simulink model "Sim_exercise2"  (R2016a)
settings: Solver=ode45  SolverMode=SingleTasking  StartTime=0.0  StopTime=10.0  RelTol=1e-3
values from neighbouring files (symbols this model uses):
  A = [-R/L 0 -Kemf/L; 0 0 1; Km/Jeq 0 -dm/Jeq]    [Exercise_1.m]    (also in Exercise_3.m = [0 1; 0 -(dm/Jeq + Km*Kemf/(R*Jeq))])
  B = [1/L; 0; 0]    [Exercise_1.m]    (also in Exercise_3.m = [0; Km/(R*Jeq)])
  C = [0 1/n 0; 0 0 1/n]    [Exercise_1.m]    (also in Exercise_3.m = [1/n 0; 0 1/n])
  D = [0; 0]    [Exercise_1.m]    (also in Exercise_3.m)
  dm = 3.8E-6    (= 3.8e-06)    [Exercise_1.m]    (also in Exercise_3.m)
  Jeq = Jm + (J1+J2)/(n^2)    (= 2.186e-06)    [Exercise_1.m]    (also in Exercise_3.m)
  Kemf = 137*2*pi/60    (= 14.3466064514)    [Exercise_1.m]    (also in Exercise_3.m = 0.0697028947848)
  Km = 69.7E-3    (= 0.0697)    [Exercise_1.m]    (also in Exercise_3.m)
  n = 5    [Exercise_1.m]    (also in Exercise_3.m)
  R = 112    [Exercise_1.m]    (also in Exercise_3.m)
undefined symbols (not defined in the file or in its folder): A1, B1, C1, D1
settings Model: Creator=sofianh  LastModifiedBy=es2lab2
settings DataIOCC: LimitDataPoints=on  SaveFormat=Array
settings OptimizationCC: BlockReduction=off  BooleanDataType=off
settings DebuggingCC: SaveWithParameterizedLinksMsg=none  UnderspecifiedInitializationDetection=Classic  MergeDetectMultiDrivingBlocksExec=none  SignalResolutionControl=TryResolveAllWithWarning  AllowSymbolicDim=off
settings HardwareCC: ProdBitPerPointer=32  ProdLargestAtomicFloat=None  ProdIntDivRoundTo=Undefined  ProdEndianess=Unspecified  ProdWordSize=32  ProdHWDeviceType=32-bit Generic  TargetUnknown=on
settings ModelReferenceCC: PropagateSignalLabelsOutOfModel=off
settings ConfigComp: CovModelRefEnable=Off  CovSFcnEnable=off

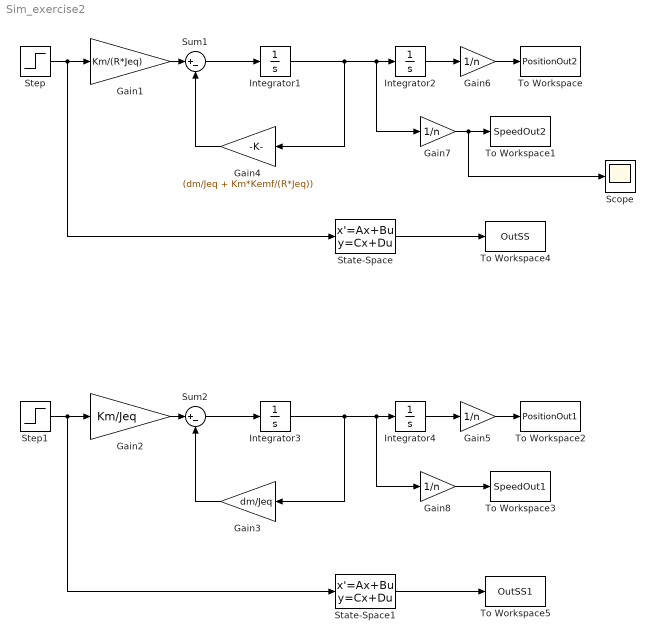
== system Sim_exercise2 ==
  Gain1 : Gain  Gain=Km/(R*Jeq)
  Gain2 : Gain  Gain=Km/Jeq
  Gain3 : Gain  Gain=dm/Jeq
  Gain4 : Gain  Gain=(dm/Jeq + Km*Kemf/(R*Jeq))
  Gain{5..8} (4 alike) : Gain  Gain=1/n
  Integrator{1..4} (4 alike) : Integrator
  Scope : Scope
  State-Space : StateSpace  A=A  B=B  C=C  D=D  X0=0  ContinuousStateAttributes='Position'
  State-Space1 : StateSpace  A=A1  B=B1  C=C1  D=D1  X0=0  ContinuousStateAttributes='Position'
  Step : Step  Time=0  After=6  SampleTime=0
  Step1 : Step  Time=0  SampleTime=0
  Sum1 : Sum  Inputs=|+-
  Sum2 : Sum  Inputs=|+-
  To Workspace : ToWorkspace  VariableName=PositionOut2  SaveFormat=Structure With Time  SampleTime=-1
  To Workspace1 : ToWorkspace  VariableName=SpeedOut2  SaveFormat=Structure With Time  SampleTime=-1
  To Workspace2 : ToWorkspace  VariableName=PositionOut1  SaveFormat=Structure With Time  SampleTime=-1
  To Workspace3 : ToWorkspace  VariableName=SpeedOut1  SaveFormat=Structure With Time  SampleTime=-1
  To Workspace4 : ToWorkspace  VariableName=OutSS  SaveFormat=Structure With Time  SampleTime=-1
  To Workspace5 : ToWorkspace  VariableName=OutSS1  SaveFormat=Structure With Time  SampleTime=-1
  wires:
  State-Space/1 -> To Workspace4/1
  Step/1 -> Gain1/1, State-Space/1
  Sum1/1 -> Integrator1/1
  Integrator1/1 -> Gain4/1, Gain7/1, Integrator2/1
  Gain4/1 -> Sum1/2
  Integrator2/1 -> Gain6/1
  Gain6/1 -> To Workspace/1
  Gain7/1 -> Scope/1, To Workspace1/1
  Gain1/1 -> Sum1/1
  State-Space1/1 -> To Workspace5/1
  Step1/1 -> Gain2/1, State-Space1/1
  Sum2/1 -> Integrator3/1
  Integrator3/1 -> Gain3/1, Gain8/1, Integrator4/1
  Gain3/1 -> Sum2/2
  Integrator4/1 -> Gain5/1
  Gain5/1 -> To Workspace2/1
  Gain8/1 -> To Workspace3/1
  Gain2/1 -> Sum2/1
